simulink model "H2_control_2dof"  (R2023b)
settings: Solver=VariableStepAuto  StartTime=0.0  StopTime=Tend_slk  RelTol=1e-3
values from neighbouring files (symbols this model uses):
  K = [-0.159911102936  -0.15905928214  -0.162463393941  -0.157973513938; -0.159068940993  -0.159920301985  -0.158265834611  -0.162753300399]    [K_H2_2dof.mat]
  Kd11 = 0.0004126    [main_H2_2dof.m]
  Kd22 = 0.0004141    [main_H2_2dof.m]
  Ki11 = 0.001599    [main_H2_2dof.m]
  Ki22 = 0.001599    [main_H2_2dof.m]
  Kp11 = 0.001625    [main_H2_2dof.m]
  Kp22 = 0.001628    [main_H2_2dof.m]
  param = [Ixx;Iyy;Izz;l;k1;k2;k3;k4;b;m]    [main_H2_2dof.m]
  Ts_slk = 0.01    [main_H2_2dof.m]
  x0 = [1;1;0;0]*0.01    [main_H2_2dof.m]
  x_des = [1;1;0;0]    [main_H2_2dof.m]
libraries: cstblocks x2, slpidlib x2
settings Model: Creator=asus  LastModifiedBy=asus
settings OptimizationCC: ReuseModelBlockBuffer=off

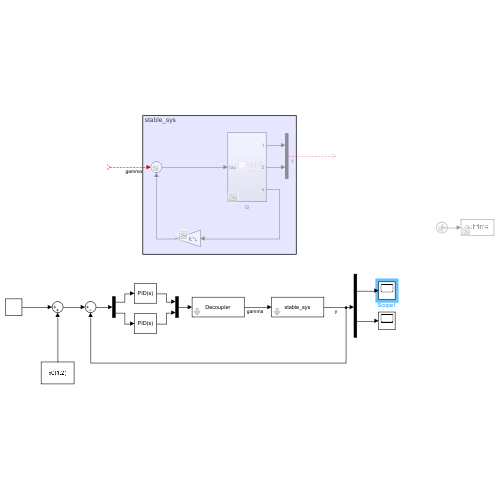
[thumbnail: Simulink's stored preview of the top-level diagram]
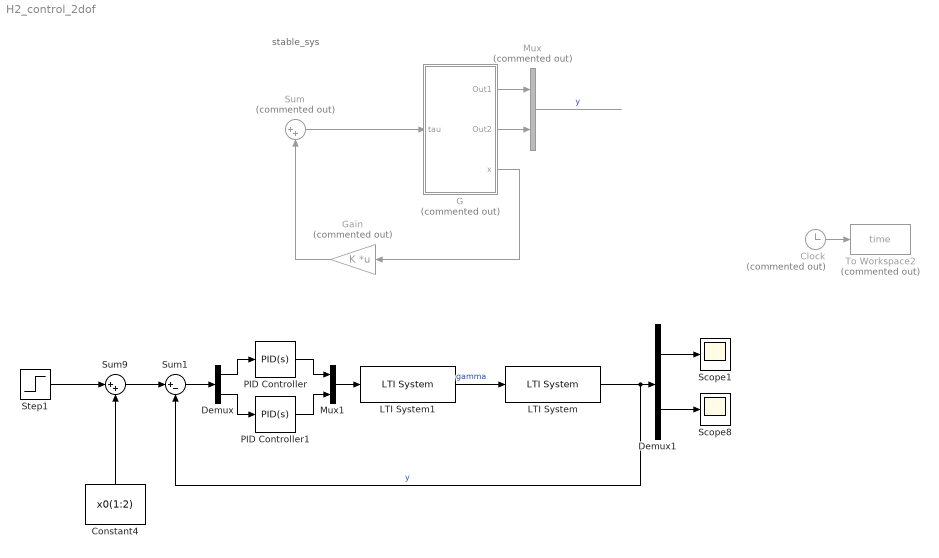
== system H2_control_2dof ==
  note: stable_sys
  Clock : Clock  Commented=on
  Constant4 : Constant  Value=x0(1:2)  SampleTime=Ts_slk
  Demux : Demux  Outputs=2
  Demux1 : Demux  Outputs=2
  G : Subsystem  Commented=on
  Gain : Gain  Commented=on  Gain=K  Multiplication=Matrix(K*u)
  LTI System : cstblocks/LTI System  sys=stable_sys  IC=[]  PadeOrder=0
  LTI System1 : cstblocks/LTI System  sys=Decoupler  IC=[]  PadeOrder=0
  Mux : Mux  Commented=on  Inputs=2
  Mux1 : Mux  Inputs=2
  PID Controller : slpidlib/PID Controller  Controller=PID  Form=Parallel  TimeDomain=Continuous-time  UseExternalTs=off  SampleTime=Ts_slk  IntegratorMethod=Forward Euler  FilterMethod=Forward Euler  ControllerParametersSource=internal  P=Kp11  I=Ki11  UseKiTs=off  D=Kd11  N=100  UseFilter=on  TunerSelectOption=Transfer Function Based (PID Tuner App)  InitialConditionSource=internal  InitialConditionForIntegrator=0  InitialConditionForFilter=0  DifferentiatorICPrevScaledInput=0  ExternalReset=none  TrackingMode=off  Kt=1  LimitOutput=off  SatLimitsSource=internal  UpperSaturationLimit=inf  LowerSaturationLimit=-inf  LinearizeAsGain=on  AntiWindupMode=none  Kb=1  LimitIntegrator=off  UpperIntegratorSaturationLimit=inf  LowerIntegratorSaturationLimit=-inf  POutMin=[]  POutMax=[]  IOutMin=[]  IOutMax=[]  DOutMin=[]  DOutMax=[]  NOutMin=[]  NOutMax=[]  SumOutMin=[]  SumOutMax=[]  SaturationOutMin=[]  SaturationOutMax=[]  PParamMin=[]  PParamMax=[]  IParamMin=[]  IParamMax=[]  DParamMin=[]  DParamMax=[]  NParamMin=[]  NParamMax=[]  KbParamMin=[]  KbParamMax=[]  KtParamMin=[]  KtParamMax=[]  KbOutMin=[]  KbOutMax=[]  KtOutMin=[]  KtOutMax=[]  IntegratorOutMin=[]  IntegratorOutMax=[]  FilterOutMin=[]  FilterOutMax=[]  SumI1OutMin=[]  SumI1OutMax=[]  SumI2OutMin=[]  SumI2OutMax=[]  SumI3OutMin=[]  SumI3OutMax=[]  SumI4OutMin=[]  SumI4OutMax=[]  SumDOutMin=[]  SumDOutMax=[]  DifferentiatorOutMin=[]  DifferentiatorOutMax=[]  FilterDiffOutCoefMin=[]  FilterDiffOutCoefMax=[]  ReciprocalOutMin=[]  ReciprocalOutMax=[]  SumDenOutMin=[]  SumDenOutMax=[]  SumNumOutMin=[]  SumNumOutMax=[]  DivideOutMin=[]  DivideOutMax=[]  UdiffTsProdOutMin=[]  UdiffTsProdOutMax=[]  NTsProdOutMin=[]  NTsProdOutMax=[]  UintegralTsProdOutMin=[]  UintegralTsProdOutMax=[]  UngainTsProdOutMin=[]  UngainTsProdOutMax=[]  ClampingZeroOutDataTypeStr=Inherit: Inherit via back propagation  ClampingZeroOutMin=[]  ClampingZeroOutMax=[]  FilterDenConstantOutDataTypeStr=Inherit: Inherit via back propagation  FilterDenConstantOutMin=[]  FilterDenConstantOutMax=[]  PCopyOutDataTypeStr=Inherit: Inherit via back propagation  PCopyOutMin=[]  PCopyOutMax=[]  NCopyOutDataTypeStr=Inherit: Inherit via back propagation  NCopyOutMin=[]  NCopyOutMax=[]  IntegratorContinuousStateAttributes=''  IntegratorStateMustResolveToSignalObject=off  IntegratorRTWStateStorageClass=Auto  FilterContinuousStateAttributes=''  FilterStateMustResolveToSignalObject=off  FilterRTWStateStorageClass=Auto  ParallelPVariant=InternalParameters  IdealPVariant=Disabled  IVariant=InternalParameters  DVariant=InternalParameters  IntegratorVariant=Continuous  SatVariant=Disabled  AWVariant=Passthrough  PCopyVariant=Disabled  TRVariant=Disabled  FdbkBlocksVariant=Forward  IdealPFdbkVariant=Disabled  SatFdbkVariant=Disabled  DerivativeFilterVariant=ContFilter  NVariant=InternalParameters  NCopyVariant=Disabled  FilterICVariant=InternalICsFilter  IntegratorICVariant=InternalICs  ExternalResetVariant=Disabled  TRSumVariant=Passthrough  SumFdbkVariant=Disabled  SumVariant=Sum_PID  TsampFilterVariant=InternalTs  TsampNgainVariant=Passthrough  TsampIntegralVariant=Disabled_SignalSpec  ExternalSaturationOutDataTypeStr=Inherit: Same as second input
  PID Controller1 : slpidlib/PID Controller  Controller=PID  Form=Parallel  TimeDomain=Continuous-time  UseExternalTs=off  SampleTime=Ts_slk  IntegratorMethod=Forward Euler  FilterMethod=Forward Euler  ControllerParametersSource=internal  P=Kp22  I=Ki22  UseKiTs=off  D=Kd22  N=100  UseFilter=on  TunerSelectOption=Transfer Function Based (PID Tuner App)  InitialConditionSource=internal  InitialConditionForIntegrator=0  InitialConditionForFilter=0  DifferentiatorICPrevScaledInput=0  ExternalReset=none  TrackingMode=off  Kt=1  LimitOutput=off  SatLimitsSource=internal  UpperSaturationLimit=inf  LowerSaturationLimit=-inf  LinearizeAsGain=on  AntiWindupMode=none  Kb=1  LimitIntegrator=off  UpperIntegratorSaturationLimit=inf  LowerIntegratorSaturationLimit=-inf  POutMin=[]  POutMax=[]  IOutMin=[]  IOutMax=[]  DOutMin=[]  DOutMax=[]  NOutMin=[]  NOutMax=[]  SumOutMin=[]  SumOutMax=[]  SaturationOutMin=[]  SaturationOutMax=[]  PParamMin=[]  PParamMax=[]  IParamMin=[]  IParamMax=[]  DParamMin=[]  DParamMax=[]  NParamMin=[]  NParamMax=[]  KbParamMin=[]  KbParamMax=[]  KtParamMin=[]  KtParamMax=[]  KbOutMin=[]  KbOutMax=[]  KtOutMin=[]  KtOutMax=[]  IntegratorOutMin=[]  IntegratorOutMax=[]  FilterOutMin=[]  FilterOutMax=[]  SumI1OutMin=[]  SumI1OutMax=[]  SumI2OutMin=[]  SumI2OutMax=[]  SumI3OutMin=[]  SumI3OutMax=[]  SumI4OutMin=[]  SumI4OutMax=[]  SumDOutMin=[]  SumDOutMax=[]  DifferentiatorOutMin=[]  DifferentiatorOutMax=[]  FilterDiffOutCoefMin=[]  FilterDiffOutCoefMax=[]  ReciprocalOutMin=[]  ReciprocalOutMax=[]  SumDenOutMin=[]  SumDenOutMax=[]  SumNumOutMin=[]  SumNumOutMax=[]  DivideOutMin=[]  DivideOutMax=[]  UdiffTsProdOutMin=[]  UdiffTsProdOutMax=[]  NTsProdOutMin=[]  NTsProdOutMax=[]  UintegralTsProdOutMin=[]  UintegralTsProdOutMax=[]  UngainTsProdOutMin=[]  UngainTsProdOutMax=[]  ClampingZeroOutDataTypeStr=Inherit: Inherit via back propagation  ClampingZeroOutMin=[]  ClampingZeroOutMax=[]  FilterDenConstantOutDataTypeStr=Inherit: Inherit via back propagation  FilterDenConstantOutMin=[]  FilterDenConstantOutMax=[]  PCopyOutDataTypeStr=Inherit: Inherit via back propagation  PCopyOutMin=[]  PCopyOutMax=[]  NCopyOutDataTypeStr=Inherit: Inherit via back propagation  NCopyOutMin=[]  NCopyOutMax=[]  IntegratorContinuousStateAttributes=''  IntegratorStateMustResolveToSignalObject=off  IntegratorRTWStateStorageClass=Auto  FilterContinuousStateAttributes=''  FilterStateMustResolveToSignalObject=off  FilterRTWStateStorageClass=Auto  ParallelPVariant=InternalParameters  IdealPVariant=Disabled  IVariant=InternalParameters  DVariant=InternalParameters  IntegratorVariant=Continuous  SatVariant=Disabled  AWVariant=Passthrough  PCopyVariant=Disabled  TRVariant=Disabled  FdbkBlocksVariant=Forward  IdealPFdbkVariant=Disabled  SatFdbkVariant=Disabled  DerivativeFilterVariant=ContFilter  NVariant=InternalParameters  NCopyVariant=Disabled  FilterICVariant=InternalICsFilter  IntegratorICVariant=InternalICs  ExternalResetVariant=Disabled  TRSumVariant=Passthrough  SumFdbkVariant=Disabled  SumVariant=Sum_PID  TsampFilterVariant=InternalTs  TsampNgainVariant=Passthrough  TsampIntegralVariant=Disabled_SignalSpec  ExternalSaturationOutDataTypeStr=Inherit: Same as second input
  Scope1 : Scope
  Scope8 : Scope
  Step1 : Step  After=x_des(1:2)*30*pi/180  SampleTime=Ts_slk
  Sum : Sum  Commented=on  Inputs=|++
  Sum1 : Sum  Inputs=|+-
  Sum9 : Sum  Inputs=|++
  To Workspace2 : ToWorkspace  Commented=on  VariableName=time  SampleTime=Ts_slk
      settings: Save2DSignal=2-D array (concatenate along first dimension)
  wires:
  Clock/1 -> To Workspace2/1
  Step1/1 -> Sum9/1
  Sum9/1 -> Sum1/1
  Constant4/1 -> Sum9/2
  Demux1/1 -> Scope1/1
  Demux1/2 -> Scope8/1
  LTI System/1 -> Sum1/2, Demux1/1  "y"
  ? -> Sum/1  "gamma"
  G/3(x) -> Gain/1
  Sum/1 -> G/1("tau ")
  G/1(Out1) -> Mux/1
  Gain/1 -> Sum/2
  G/2(Out2) -> Mux/2
  Mux/1 -> ?  "y"
  LTI System1/1 -> LTI System/1  "gamma"
  Mux1/1 -> LTI System1/1
  PID Controller/1 -> Mux1/1
  PID Controller1/1 -> Mux1/2
  Demux/1 -> PID Controller/1
  Sum1/1 -> Demux/1
  Demux/2 -> PID Controller1/1

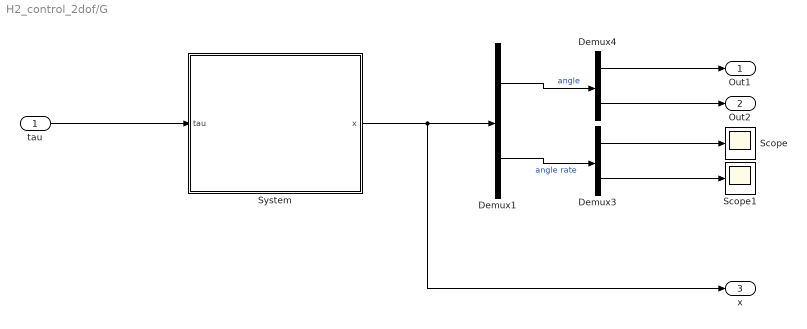
== system H2_control_2dof/G ==
  "tau " : Inport
  Demux1 : Demux  Outputs=2
  Demux3 : Demux  Outputs=2
  Demux4 : Demux  Outputs=2
  Scope : Scope
  Scope1 : Scope
  System : Subsystem
  Out1 : Outport
  Out2 : Outport  Port=2
  x : Outport  Port=3
  wires:
  System/1(x) -> x/1, Demux1/1
  Demux3/1 -> Scope/1
  Demux4/1 -> Out1/1
  Demux1/1 -> Demux4/1  "angle"
  Demux1/2 -> Demux3/1  "angle rate"
  Demux3/2 -> Scope1/1
  Demux4/2 -> Out2/1
  "tau "/1 -> System/1("tau ")

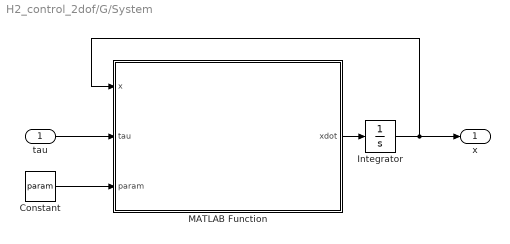
== system H2_control_2dof/G/System ==
  "tau " : Inport
  Constant : Constant  Value=param
  Integrator : Integrator  InitialCondition=x0
  MATLAB Function : MATLAB Function  TreatAsAtomicUnit=on
  x : Outport
  wires:
  Integrator/1 -> MATLAB Function/1(x), x/1
  MATLAB Function/1(xdot) -> Integrator/1
  "tau "/1 -> MATLAB Function/2(tau)
  Constant/1 -> MATLAB Function/3(param)

== matlab function H2_control_2dof/G/System/MATLAB Function ==
  data: x input; tau input; xdot output; param input
function xdot =quadcopter(x,tau,param)
% Inputs:
%           x       (model state)
%           tau     (torque)           
%           param   (model parameters)
%
% Outputs:  x_dot  (derivative of the state with respect to time)

% Parameters
g        =       9.81;           %  gravity acceleration (m/s^2)
Ixx      =       param(1,1);     %  moment of inertia 
Iyy      =       param(2,1);     %  moment of inertia
Izz      =       param(3,1);     %  moment of inertia 

% States
phi      =       x(1,1);     %  roll angle (rad)
theta    =       x(2,1);     %  pitch angle (rad)
phi_dot  =       x(3,1);     %  roll rate (rad/s)
theta_dot=       x(4,1);     %  pitch rate (rad/s)

cph         =       cos(phi);
cth         =       cos(theta);
sph         =       sin(phi);
sth         =       sin(theta);

% torques
tau_1    =       tau(1,1);   %  roll torque 
tau_2    =       tau(2,1);   %  pitch torque  

% Coriolis matrix
C11=  0;
C12= (Iyy)*(theta_dot*cph*sph);
C21= (Iyy)*(theta_dot*cph*sph);
C22= 0;

C  = [C11 C12;
      C21 C22];

% Inertia matrix
J11= Ixx;
J12= 0;
J21= 0;
J22= Iyy*cph^2;

J  = [J11 J12;
     J21 J22];

%% Model Equation 
invJ = [ J22/(J11*J22 - J12*J21), -J12/(J11*J22 - J12*J21);
        -J21/(J11*J22 - J12*J21),  J11/(J11*J22 - J12*J21)];

xdot        = zeros(4,1);
xdot(1:2,1) = x(3:4,1);
xdot(3:4,1) = invJ*(tau - C*x(3:4,1));
